simulink model "mogen_SMU"  (Simulink 9.2)
settings: Solver=ode4  StartTime=0.0  StopTime=inf  FixedStep=model_sample_time  RelTol=1e-3
undefined symbols (not defined in the file): magnitude, model_sample_time
libraries: utils x4, simulink x2
(part 4 of 4)

== matlab function move2pose1/p2p/fs_function ==
  data: t input double; T input double; psi input double; time_factor output double; Gamma input double; Theta input double; k input double; interpoly input double
function time_factor = fs_function_time(t, T, psi, Gamma, Theta, k, interpoly)
%FS_FUNCTION_TIME computes the scaling factor for the next timestep. It is 
% similar to equotation (14) of the reference, except that Theta adds a
% parameter for smoother decline and it allows a slower decline. This is
% achieved by the introduction of time t and setting a duration T for the
% adaption. Phi function underneath is similar to (16) of the reference.
%
% Reference:
% [1] S. Haddadin, A. Albu-Schäffer, A. De Luca, and G. Hirzinger, 
% "Collision detection and reaction: A contribution to safe physical 
% human-robot interaction,” International Conference on Intelligent Robots 
% and Systems, pp. 3356–3363, 2008.
%
% Input variables
% t           = Current runtime
% T           = Duration of adaption
% psi         = Scaling factor for time; 0=No scaling; Theta=stop;
%               >Theta+Gamma = revert motion
% Gamma       = Optional dead-zone between stop and reverting motion (set 0
%               for deactivation)
% Theta       = Optional smoothness or strechting(set 1 for deactivation) 
% k           = speed factor for pushing back; 1=deactivated; the higher 
%               the faster the reverting motion
% interpoly   = Which interpolation to use
%
% Output variables
% time_factor = Factor for scaling the next time increment; 0=Stop motion;
%               1= Normal speed; negative values = revert motion
    
%% Initialize persistent variables for adaption motion
persistent psi_1 adpt ti psi_i
if isempty(psi_1)
    psi_1 = psi;    %remembers the psi from last run
end
if isempty(adpt)
    adpt = false;   %stores if an adaption motion is activated
end
if isempty(ti)
    ti = 0;         %Initial time step for adaption motion
end
if isempty(psi_i)
    psi_i = 0;      %Initial psi for adaption motion
end

% needed to delay tanhlog with one timestep
tanhlog_delay = 0;

%% This If runs only for one timestep!!!
% If current psi is unequal to old one 
% Not directly at the beginning
% Dont start new while a adaption is still running, to prevent reset of
%   initial values
if abs(psi-psi_1)>1e-6 && t>0.001 && adpt==false                          
    adpt=true;          % Activate adaption
    ti=t;               % Set initial timestep to current step

    %%% inital set of position, velo, acceleration for adaption motion 
    psi_i = psi_1;
    tanhlog_delay = 1;    
end

%% If adaption motion needed
if adpt == true 

    %%% calculate the adaption psi, which takes time from ti to
    % ti+T. t is the current runtime, _i initial values, _f final
    % values, _m maximum values

    switch interpoly
        case 0
            adpt=false;         %no adatption  
            psi_adpt = psi;
        case 1
            if tanhlog_delay == 1
                psi_adpt = psi_i;
                tanhlog_delay = 0;
            else
                psi_adpt = tanhlog(t-ti,T,psi_i,psi);  %tanhlog
            end
        case 2
            psi_adpt = cosine(t-ti,T,psi_i,psi);   %Cosine version
        case 3
            psi_adpt = poly3(t-ti,T,psi_i,psi);    %poly3
        case 4
            psi_adpt = poly4(t-ti,T,psi_i,psi);    %poly4
        case 5
            psi_adpt = poly5(t-ti,T,psi_i,psi);    %poly5 
        case 6
            psi_adpt = poly6(t-ti,T,psi_i,psi);    %poly6 
        case 7
            psi_adpt = poly7(t-ti,T,psi_i,psi);    %poly7
        case 10
            psi_adpt = tanhmean(t-ti,T,psi_i,psi);    %tanhmean 
        otherwise
            error('Unknown adaption motion');   %rest
    end

    % This computes the time_factor with the standard fs_function, if there is
    % an adaption running
    time_factor = fs_function_lin(psi_adpt, Gamma, Theta, k);

    %if time is equal than the finish time => adaption motion is complete
    %But it is aborted one timestep earlier, since the finish timestep
    %is already computed correctly by the standard interpolator.
    if t>=(ti+T-0.001)  
        adpt=false;     %If adaption finished => reset
    end
    
else %% time_factor without adaption  
    % This computes the time_factor with the standard fs_function, if there is
    % no adaption
    % Linear decline needed here, since smoothness is in time
    time_factor = fs_function_lin(psi, Gamma, Theta, k);
end

psi_1 = psi;  %remember current psi

end

function time_factor = fs_function(psi, Gamma, Theta, k)
%FS_FUNCTION computes the scaling factor for the next timestep. It is 
% similar to equotation (14) of the reference, except that Theta adds a
% parameter for smoother decline. Phi function underneath is similar to
% (16) of the reference.
%
% Reference:
% [1] S. Haddadin, A. Albu-Schäffer, A. De Luca, and G. Hirzinger, 
% "Collision detection and reaction: A contribution to safe physical 
% human-robot interaction,” International Conference on Intelligent Robots 
% and Systems, pp. 3356–3363, 2008.

% Input variables
% psi         = Scaling factor for time; 0=No scaling; Theta=stop;
%               >Theta+Gamma = revert motion
% Gamma       = Optional dead-zone between stop and reverting motion (set 0
%               for deactivation)
% Theta       = Optional smoothness or strechting(set 1 for deactivation) 
% k           = speed factor for pushing back; 1=deactivated; the higher 
%               the faster the reverting motion

% Output variables
% time_factor = Factor for scaling the next time increment; 0=Stop motion;
%               1= Normal speed; negative values = revert motion
       
time_factor = 0;
if 0 <= psi && psi < Theta    %Equ. (14)
    time_factor = phi(psi, Theta);
elseif Theta <= psi && psi <= Theta+Gamma
    time_factor = 0;
elseif Theta+Gamma < psi && psi <= 2*Theta+Gamma
    time_factor = k*phi(psi-Theta-Gamma, Theta)-k;
elseif 2*Theta+Gamma < psi
    time_factor = -k;
else
    error('Trajectory scaling - fs_function: psi wrong (e.g. psi<0)');
end

end

function [psi_smooth] = phi(psi, Theta)
%PHI computes formular (16); smoother decline of factor
%
% Reference:
% [1] S. Haddadin, A. Albu-Schäffer, A. De Luca, and G. Hirzinger, 
% "Collision detection and reaction: A contribution to safe physical 
% human-robot interaction,” International Conference on Intelligent Robots 
% and Systems, pp. 3356–3363, 2008.
%
% Input variables
% psi     = Scaling factor for time (could be vector to here)
% Theta   = Optional smoothness or strechting(set 1 for deactivation)
%
% Output variables
% psi_smooth = smoother psi value

psi_smooth = 0.5.*(ones(size(psi))+cos((1/Theta)*pi.*psi)); %Equ. (16)

end

function time_factor = fs_function_lin(psi, Gamma, Theta, k)
%FS_FUNCTION_LIN computes the scaling factor for the next timestep. It is 
% similar to equotation (14) of the reference, except that Theta adds a
% parameter for smoother decline. Phi function underneath is linear decline
%
% Reference:
% [1] S. Haddadin, A. Albu-Schäffer, A. De Luca, and G. Hirzinger, 
% "Collision detection and reaction: A contribution to safe physical 
% human-robot interaction,” International Conference on Intelligent Robots 
% and Systems, pp. 3356–3363, 2008.

% Input variables
% psi         = Scaling factor for time; 0=No scaling; Theta=stop;
%               >Theta+Gamma = revert motion
% Gamma       = Optional dead-zone between stop and reverting motion (set 0
%               for deactivation)
% Theta       = Optional smoothness or strechting(set 1 for deactivation) 
% k           = speed factor for pushing back; 1=deactivated; the higher 
%               the faster the reverting motion

% Output variables
% time_factor = Factor for scaling the next time increment; 0=Stop motion;
%               1= Normal speed; negative values = revert motion
       
time_factor = 0;
if 0 <= psi && psi < Theta    %Equ. (14)
    time_factor = lin(psi, Theta);
elseif Theta <= psi && psi <= Theta+Gamma
    time_factor = 0;
elseif Theta+Gamma < psi && psi <= 2*Theta+Gamma
    time_factor = k*lin(psi-Theta-Gamma, Theta)-k;
elseif 2*Theta+Gamma < psi
    time_factor = -k;
else
    error('Trajectory scaling - fs_function: psi wrong (e.g. psi<0)');
end

end

function [psi_smooth] = lin(psi, Theta)
%LIN computes linear decline of factor. selfmade
%
% Input variables
% psi     = Scaling factor for time (could be vector to here)
% Theta   = Optional smoothness or strechting(set 1 for deactivation)
%
% Output variables
% psi_smooth = smoother psi value

psi_smooth = 1-(psi/Theta);

end

function [psi] = tanhlog(t,T,psi_i,psi_f)
%TANHLOG computes a 2 tanh-log trajectories between initial (_i) 
%values and final (_f) values of psi. The first goes to a virtual line in 
%the middle and the second back to d_psi_f=0.
%taken from Internet

psi_mean = (psi_f+psi_i)/2;             % calculate mean value of inital and final value
virt_slope = (4*psi_mean-4*psi_i)/T;    % define slope of virtual line 
virt_shift = psi_mean - virt_slope*T/2; % compute the shift of the virtual line

if t<=T/2 %first part for inital to virtual
    a = 0;         
    b = psi_i; 
    c = virt_slope;
    d = virt_shift;
    k = d-b;

    x = (a*t+b-c*t-d+k)/(2*k);
    w = (tanh(((log(1-x))^2-(log(x))^2)/3)+1)/2;
    p = tanh((log(2-x)-log(x))*(1-(1/sqrt(2))*(log(2-x)+log(x))))+2*x-1;
    q = tanh((log(x+1)-log(1-x))*(1-(1/sqrt(2))*(log(1-x)+log(x+1))));
    s = p*(1-w)+q*w;

    psi = k*s+c*t+d-k;
else    %second part from virtual to final
    a = virt_slope;
    b = virt_shift;
    c = 0;     
    d = psi_f; 
    k = (d-b)*(1/3); %k has to be computed a bit different. Math...

    x = (a*t+b-c*t-d+k)/(2*k);
    w = (tanh(((log(1-x))^2-(log(x))^2)/3)+1)/2;
    p = tanh((log(2-x)-log(x))*(1-(1/sqrt(2))*(log(2-x)+log(x))))+2*x-1;
    q = tanh((log(x+1)-log(1-x))*(1-(1/sqrt(2))*(log(1-x)+log(x+1))));
    s = p*(1-w)+q*w;

    psi = k*s+c*t+d-k;
end

end

function [psi] = cosine(t,T,psi_i,psi_f)
%COSINE computes a cosine trajectory between initial (_i) 
%values and final (_f) values of psi. t is the time since ti; T the
%duration
   
psi = 0.5*(psi_i+psi_f) + 0.5*(psi_i-psi_f)*cos((pi/T)*t);

end

function [psi] = poly3(t,T,psi_i,psi_f)
%POLY3 computes a polynomial trajectory of degree 3 between initial (_i) 
%values and final (_f) values of psi. selfmade with poly_calc

d_psi_i = 0; %with poly3 an adaption to the velocity of the change of psi would be possible
d_psi_f = 0;

a = [...
 conj(psi_i)
 conj(d_psi_i)
 (3*conj(psi_f))/T^2 - (2*conj(d_psi_i))/T - conj(d_psi_f)/T - (3*conj(psi_i))/T^2
 conj(d_psi_f)/T^2 + conj(d_psi_i)/T^2 - (2*conj(psi_f))/T^3 + (2*conj(psi_i))/T^3];

psi = a(1)+a(2)*t+a(3)*t^2+a(4)*t^3;

end

function [psi] = poly4(t,T,psi_i,psi_f)
%POLY4 computes a polynomial trajectory of degree 4 between initial (_i) 
%values and final (_f) values of psi. selfmade with poly_calc

d_psi_i = 0; %with poly4 an adaption to the velocity of the change of psi would be possible
d_psi_f = 0;
dd_psi_f = 0;

a = [...
                                                                                                    conj(psi_i)
                                                                                                  conj(d_psi_i)
       conj(dd_psi_f)/2 - (3*conj(d_psi_f))/T - (3*conj(d_psi_i))/T + (6*conj(psi_f))/T^2 - (6*conj(psi_i))/T^2
   (5*conj(d_psi_f))/T^2 + (3*conj(d_psi_i))/T^2 - conj(dd_psi_f)/T - (8*conj(psi_f))/T^3 + (8*conj(psi_i))/T^3
 conj(dd_psi_f)/(2*T^2) - conj(d_psi_i)/T^3 - (2*conj(d_psi_f))/T^3 + (3*conj(psi_f))/T^4 - (3*conj(psi_i))/T^4];

psi = a(1)+a(2)*t+a(3)*t^2+a(4)*t^3+a(5)*t^4;

end

function [psi] = poly5(t,T,psi_i,psi_f)
%POLY4 computes a polynomial trajectory of degree 4 between initial (_i) 
%values and final (_f) values of psi. selfmade with poly_calc

d_psi_i = 0; %with poly4 an adaption to the velocity of the change of psi would be possible
d_psi_f = 0;
dd_psi_i = 0;
dd_psi_f = 0;

a = [...
                                                                                                                                   conj(psi_i)
                                                                                                                                 conj(d_psi_i)
                                                                                                                              conj(dd_psi_i)/2
 conj(dd_psi_f)/(2*T) - (6*conj(d_psi_i))/T^2 - (4*conj(d_psi_f))/T^2 - (3*conj(dd_psi_i))/(2*T) + (10*conj(psi_f))/T^3 - (10*conj(psi_i))/T^3
 (7*conj(d_psi_f))/T^3 + (8*conj(d_psi_i))/T^3 - conj(dd_psi_f)/T^2 + (3*conj(dd_psi_i))/(2*T^2) - (15*conj(psi_f))/T^4 + (15*conj(psi_i))/T^4
   conj(dd_psi_f)/(2*T^3) - (3*conj(d_psi_i))/T^4 - (3*conj(d_psi_f))/T^4 - conj(dd_psi_i)/(2*T^3) + (6*conj(psi_f))/T^5 - (6*conj(psi_i))/T^5];

psi = a(1)+a(2)*t+a(3)*t^2+a(4)*t^3+a(5)*t^4+a(6)*t^5;

end

function [psi] = poly6(t,T,psi_i,psi_f)
%POLY6 computes a polynomial trajectory of degree 6 between initial (_i) 
%values and final (_f) values of psi. j_m is max jerk. selfmade with poly_calc

d_psi_i = 0; %with poly4 an adaption to the velocity of the change of psi would be possible
d_psi_f = 0;
dd_psi_i = 0;
dd_psi_f = 0;
j_m = 50;

a = [...
                                                                                                                                                           conj(psi_i)
                                                                                                                                                         conj(d_psi_i)
                                                                                                                                                      conj(dd_psi_i)/2
                                                                                                                                                           conj(j_m)/6
      conj(dd_psi_f)/(2*T^2) - (10*conj(d_psi_i))/T^3 - (5*conj(d_psi_f))/T^3 - (3*conj(dd_psi_i))/T^2 - conj(j_m)/(2*T) + (15*conj(psi_f))/T^4 - (15*conj(psi_i))/T^4
        (9*conj(d_psi_f))/T^4 + (15*conj(d_psi_i))/T^4 - conj(dd_psi_f)/T^3 + (4*conj(dd_psi_i))/T^3 + conj(j_m)/(2*T^2) - (24*conj(psi_f))/T^5 + (24*conj(psi_i))/T^5
 conj(dd_psi_f)/(2*T^4) - (6*conj(d_psi_i))/T^5 - (4*conj(d_psi_f))/T^5 - (3*conj(dd_psi_i))/(2*T^4) - conj(j_m)/(6*T^3) + (10*conj(psi_f))/T^6 - (10*conj(psi_i))/T^6];

psi = a(1)+a(2)*t+a(3)*t^2+a(4)*t^3+a(5)*t^4+a(6)*t^5+a(7)*t^6;

end

function [psi] = poly7(t,T,psi_i,psi_f)
%POLY6 computes a polynomial trajectory of degree 6 between initial (_i) 
%values and final (_f) values of psi. j_m is max jerk. selfmade with poly_calc

d_psi_i = 0; %with poly4 an adaption to the velocity of the change of psi would be possible
d_psi_f = 0;
dd_psi_i = 0;
dd_psi_f = 0;
ddd_psi_i = 0;
ddd_psi_f = 0;

a = [...
                                                                                                                                                                                                       conj(psi_i)
                                                                                                                                                                                                     conj(d_psi_i)
                                                                                                                                                                                                  conj(dd_psi_i)/2
                                                                                                                                                                                                 conj(ddd_psi_i)/6
           (5*conj(dd_psi_f))/(2*T^2) - (20*conj(d_psi_i))/T^3 - (15*conj(d_psi_f))/T^3 - (5*conj(dd_psi_i))/T^2 - conj(ddd_psi_f)/(6*T) - (2*conj(ddd_psi_i))/(3*T) + (35*conj(psi_f))/T^4 - (35*conj(psi_i))/T^4
                  (39*conj(d_psi_f))/T^4 + (45*conj(d_psi_i))/T^4 - (7*conj(dd_psi_f))/T^3 + (10*conj(dd_psi_i))/T^3 + conj(ddd_psi_f)/(2*T^2) + conj(ddd_psi_i)/T^2 - (84*conj(psi_f))/T^5 + (84*conj(psi_i))/T^5
 (13*conj(dd_psi_f))/(2*T^4) - (36*conj(d_psi_i))/T^5 - (34*conj(d_psi_f))/T^5 - (15*conj(dd_psi_i))/(2*T^4) - conj(ddd_psi_f)/(2*T^3) - (2*conj(ddd_psi_i))/(3*T^3) + (70*conj(psi_f))/T^6 - (70*conj(psi_i))/T^6
               (10*conj(d_psi_f))/T^6 + (10*conj(d_psi_i))/T^6 - (2*conj(dd_psi_f))/T^5 + (2*conj(dd_psi_i))/T^5 + conj(ddd_psi_f)/(6*T^4) + conj(ddd_psi_i)/(6*T^4) - (20*conj(psi_f))/T^7 + (20*conj(psi_i))/T^7];

psi = a(1)+a(2)*t+a(3)*t^2+a(4)*t^3+a(5)*t^4+a(6)*t^5+a(7)*t^6+a(8)*t^7;

end

function [psi] = tanhmean(t,T,psi_i,psi_f)
%TANHMEAN computes a tanh trajectory between initial (_i) 
%values and final (_f) values of psi. theta is the slope of the transition
%selfmade
                     
t_norm = t/T; %Normalized time necessary for this function
theta = 4;

psi = 0.5*(psi_i+psi_f) + 0.5*(psi_f-psi_i)*tanh(theta*(t_norm-0.5));

end

== matlab function move2pose1/p2p/psi_velocity ==
  data: v_desired input double; psi output double; v_safe input double
function psi  = psi_velocity(v_desired, v_safe)
%PSI_VELOCITY Computes a psi value from the comparison of two
%velocities. v_desired is the velocity the robot should move and v_safe
%sets an upper limit. The returned psi value scales down the velocity to a 
%safe value. Both values can be vectors, then the function checks the psi
%value for each dimension and returns the most restrictive psi (=highest).
%
% Input variables
% v_desired = The velocity the robot should move with
% v_safe    = The maximal velocity which is safe for this movement
%
% Output variables
% psi       = value for influencing the speed of the robot

psi = 0;
n = size(v_desired,2);  %n= dimension of velocity
psis = zeros(n,1);      %predefine vector for each dimension
for i=1:n               %Check each dimension
    psis(i) = psi_velocity_single(v_desired(i), v_safe(i));
end

psi = max(psis);        %Take most restrictive psi for all dimensions

end

function [psi_single] = psi_velocity_single(v_desired, v_safe)
%PSI_VELOCITY_SINGLE Computes a psi value from the comparison of two
%velocities. v_desired is the velocity the robot should move and v_safe
%sets an upper limit. The returned psi value scales down the velocity to a 
%safe value, if v_desired is greater than v_safe. This function compares
%only one dimension.
%
% Input variables
% v_desired  = The velocity the robot should move with
% v_safe     = The maximal velocity which is safe for this movement
%
% Output variables
% psi_single = value for influencing the speed of the robot

psi_single = 0.0;
if v_desired <= 1.0*v_safe                   %No danger
    psi_single = 0.0;                     %=> No scaling
elseif v_desired > 1.0*v_safe              %Desired velocity is dangerous
	psi_single = (1-(v_safe/v_desired));%=> Scaling of time to safe velocity
end

end
